simulink subsystem "slagEnergyBalance"  (R2024a)
settings: Solver=VariableStepAuto  StartTime=0.0  StopTime=2014080  RelTol=1e-3
undefined symbols (not defined in the file): bath_area, matte_specific_heat_capacity, slag_charge_heat_transfer_coefficient, slag_in_temperature, slag_matte_heat_transfer_coefficient, slag_specific_heat_capacity, water_specific_heat_capacity
settings Model: DataDictionary=constants.sldd  EnableAccessToBaseWorkspace=off  DefaultTestHarness=slagEnergyBalance_HarnessFromWorkspace  Creator=jason.miskin  LastModifiedBy=jason.miskin

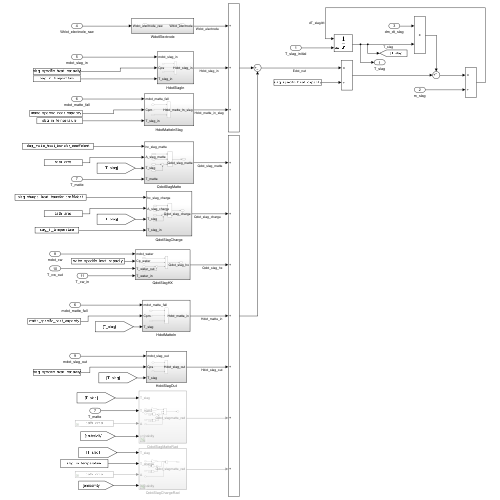
[thumbnail: Simulink's stored preview of the top-level diagram]
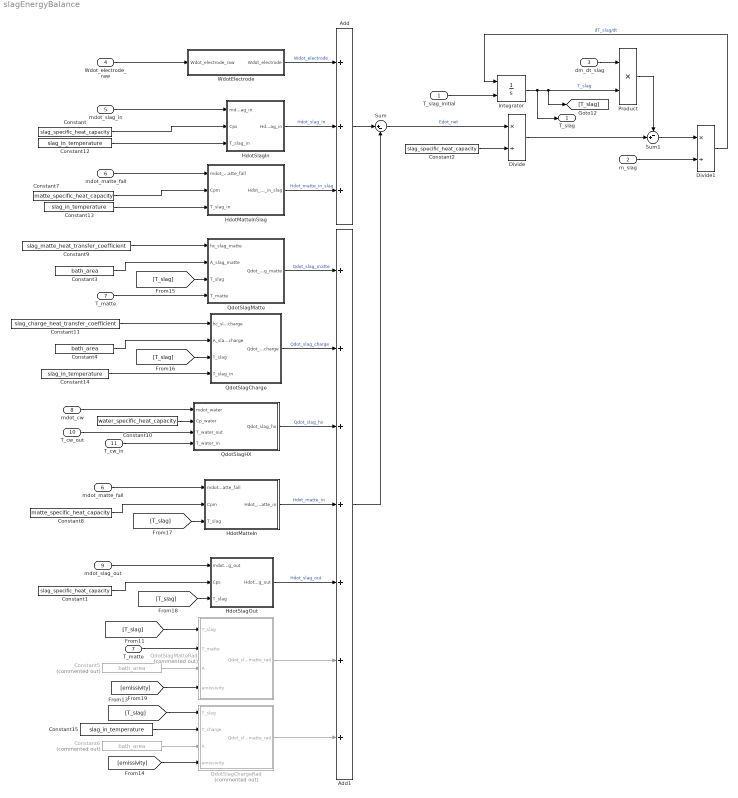
== system slagEnergyBalance ==
  T_slag_initial : Inport
  m_slag : Inport  Port=2
  dm_dt_slag : Inport  Port=3
  Wdot_electrode_raw : Inport  Port=4
  mdot_slag_in : Inport  Port=5
  mdot_matte_fall : Inport  Port=6
  T_matte : Inport  Port=7
  mdot_cw : Inport  Port=8
  mdot_slag_out : Inport  Port=9
  T_cw_out : Inport  Port=10
  T_cw_in : Inport  Port=11
  Add : Sum  Inputs=3
  Add1 : Sum  Inputs=7
  Constant : Constant  Value=slag_specific_heat_capacity
  Constant1 : Constant  Value=slag_specific_heat_capacity
  Constant10 : Constant  Value=water_specific_heat_capacity
  Constant11 : Constant  Value=slag_charge_heat_transfer_coefficient
  Constant{12..15} (4 alike) : Constant  Value=slag_in_temperature
  Constant2 : Constant  Value=slag_specific_heat_capacity
  Constant3 : Constant  Value=bath_area
  Constant4 : Constant  Value=bath_area
  Constant5 : Constant  Commented=on  Value=bath_area
  Constant6 : Constant  Commented=on  Value=bath_area
  Constant7 : Constant  Value=matte_specific_heat_capacity
  Constant8 : Constant  Value=matte_specific_heat_capacity
  Constant9 : Constant  Value=slag_matte_heat_transfer_coefficient
  Divide : Product  Inputs=*/
  Divide1 : Product  Inputs=*/
  HdotMatteIn : Subsystem
  HdotMatteInSlag : Subsystem
  HdotSlagIn : Subsystem
  HdotSlagOut : Subsystem
  Integrator : Integrator  InitialConditionSource=external
  Product : Product
  QdotSlagCharge : Subsystem
  QdotSlagChargeRad : Subsystem  Commented=on
  QdotSlagHX : Subsystem
  QdotSlagMatte : Subsystem
  QdotSlagMatteRad : Subsystem  Commented=on
  Sum : Sum  Inputs=|+-
  Sum1 : Sum  Inputs=-+|
  "T_matte " : InportShadow  Port=7
  WdotElectrode : Subsystem
  "mdot_matte_fall " : InportShadow  Port=6
  T_slag : Outport
  wires:
  WdotElectrode/1(Wdot_electrode) -> Add/1  "Wdot_electrode"
  Sum/1 -> Divide/1  "Edot_net"
  Constant/1 -> HdotSlagIn/2(Cps)
  [T_slag] -> HdotMatteIn/3(T_slag)
  Constant12/1 -> HdotSlagIn/3(T_slag_in)
  mdot_matte_fall/1 -> HdotMatteInSlag/1(mdot_matte_fall)
  T_slag_initial/1 -> Integrator/2
  Constant7/1 -> HdotMatteInSlag/2(Cpm)
  Divide/1 -> Sum1/2
  Constant3/1 -> QdotSlagMatte/2(A_slag_matte)
  mdot_slag_out/1 -> HdotSlagOut/1(mdot_slag_out)
  Divide1/1 -> Integrator/1  "dT_slag/dt"
  Constant9/1 -> QdotSlagMatte/1(hc_slag_matte)
  HdotSlagIn/1(Hdot_slag_in) -> Add/2  "Hdot_slag_in"
  dm_dt_slag/1 -> Product/1
  HdotMatteInSlag/1(Hdot_matte_in_slag) -> Add/3  "Hdot_matte_in_slag"
  HdotMatteIn/1(Hdot_matte_in) -> Add1/4  "Hdot_matte_in"
  Add/1 -> Sum/1
  QdotSlagMatte/1(Qdot_slag_matte) -> Add1/1  "Qdot_slag_matte"
  Integrator/1 -> Product/2, [T_slag], T_slag/1  "T_slag"
  Constant11/1 -> QdotSlagCharge/1(hc_slag_charge)
  m_slag/1 -> Divide1/2
  Add1/1 -> Sum/2
  Wdot_electrode_raw/1 -> WdotElectrode/1(Wdot_electrode_raw)
  QdotSlagCharge/1(Qdot_slag_charge) -> Add1/2  "Qdot_slag_charge"
  HdotSlagOut/1(Hdot_slag_out) -> Add1/5  "Hdot_slag_out"
  [T_slag] -> HdotSlagOut/3(T_slag)
  mdot_slag_in/1 -> HdotSlagIn/1(mdot_slag_in)
  Product/1 -> Sum1/1
  [T_slag] -> QdotSlagCharge/3(T_slag)
  [T_slag] -> QdotSlagMatte/3(T_slag)
  Sum1/1 -> Divide1/1
  mdot_cw/1 -> QdotSlagHX/1(mdot_water)
  QdotSlagHX/1(Qdot_slag_hx) -> Add1/3  "Qdot_slag_hx"
  T_matte/1 -> QdotSlagMatte/4(T_matte)
  Constant2/1 -> Divide/2
  Constant1/1 -> HdotSlagOut/2(Cps)
  Constant13/1 -> HdotMatteInSlag/3(T_slag_in)
  Constant14/1 -> QdotSlagCharge/4(T_slag_in)
  "mdot_matte_fall "/1 -> HdotMatteIn/1(mdot_matte_fall)
  Constant8/1 -> HdotMatteIn/2(Cpm)
  Constant4/1 -> QdotSlagCharge/2(A_slag_charge)
  T_cw_out/1 -> QdotSlagHX/3(T_water_out)
  T_cw_in/1 -> QdotSlagHX/4(T_water_in)
  Constant10/1 -> QdotSlagHX/2(Cp_water)
  Constant5/1 -> QdotSlagMatteRad/3(A)
  [T_slag] -> QdotSlagMatteRad/1(T_slag)
  "T_matte "/1 -> QdotSlagMatteRad/2(T_matte)
  Constant15/1 -> QdotSlagChargeRad/2(T_charge)
  Constant6/1 -> QdotSlagChargeRad/3(A)
  [T_slag] -> QdotSlagChargeRad/1(T_slag)
  QdotSlagMatteRad/1(Qdot_slagmatte_rad) -> Add1/6
  QdotSlagChargeRad/1(Qdot_slagmatte_rad) -> Add1/7
  [emissivity] -> QdotSlagChargeRad/4(emissivity)
  [emissivity] -> QdotSlagMatteRad/4(emissivity)

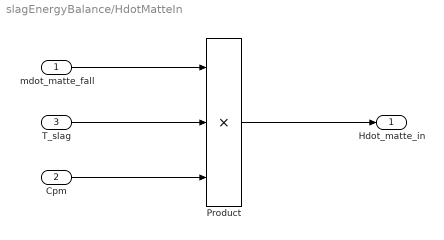
== system slagEnergyBalance/HdotMatteIn ==
  mdot_matte_fall : Inport
  Cpm : Inport  Port=2
  T_slag : Inport  Port=3
  Product : Product  Inputs=3
  Hdot_matte_in : Outport
  wires:
  T_slag/1 -> Product/2
  mdot_matte_fall/1 -> Product/1
  Product/1 -> Hdot_matte_in/1
  Cpm/1 -> Product/3

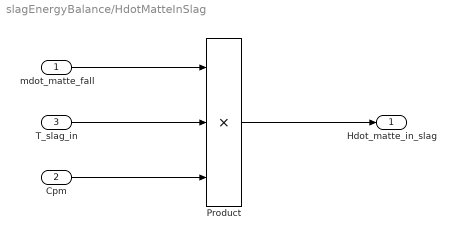
== system slagEnergyBalance/HdotMatteInSlag ==
  mdot_matte_fall : Inport
  Cpm : Inport  Port=2
  T_slag_in : Inport  Port=3
  Product : Product  Inputs=3
  Hdot_matte_in_slag : Outport
  wires:
  Cpm/1 -> Product/3
  mdot_matte_fall/1 -> Product/1
  Product/1 -> Hdot_matte_in_slag/1
  T_slag_in/1 -> Product/2

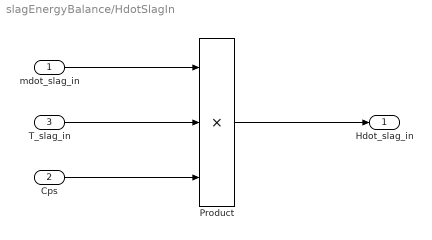
== system slagEnergyBalance/HdotSlagIn ==
  mdot_slag_in : Inport
  Cps : Inport  Port=2
  T_slag_in : Inport  Port=3
  Product : Product  Inputs=3
  Hdot_slag_in : Outport
  wires:
  Cps/1 -> Product/3
  T_slag_in/1 -> Product/2
  mdot_slag_in/1 -> Product/1
  Product/1 -> Hdot_slag_in/1

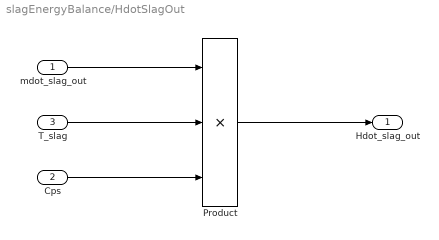
== system slagEnergyBalance/HdotSlagOut ==
  mdot_slag_out : Inport
  Cps : Inport  Port=2
  T_slag : Inport  Port=3
  Product : Product  Inputs=3
  Hdot_slag_out : Outport
  wires:
  Cps/1 -> Product/3
  mdot_slag_out/1 -> Product/1
  T_slag/1 -> Product/2
  Product/1 -> Hdot_slag_out/1

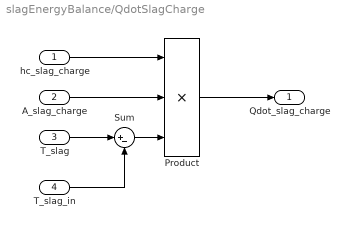
== system slagEnergyBalance/QdotSlagCharge ==
  hc_slag_charge : Inport
  A_slag_charge : Inport  Port=2
  T_slag : Inport  Port=3
  T_slag_in : Inport  Port=4
  Product : Product  Inputs=3
  Sum : Sum  Inputs=|+-
  Qdot_slag_charge : Outport
  wires:
  hc_slag_charge/1 -> Product/1
  A_slag_charge/1 -> Product/2
  T_slag/1 -> Sum/1
  T_slag_in/1 -> Sum/2
  Sum/1 -> Product/3
  Product/1 -> Qdot_slag_charge/1

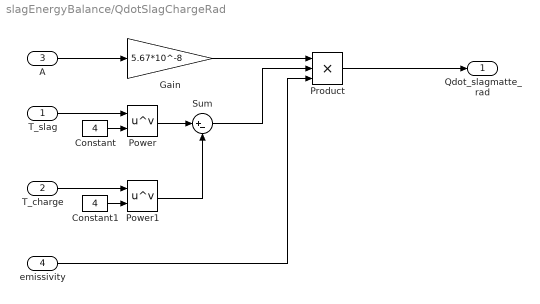
== system slagEnergyBalance/QdotSlagChargeRad ==
  T_slag : Inport
  T_charge : Inport  Port=2
  A : Inport  Port=3
  emissivity : Inport  Port=4
  Constant : Constant  Value=4
  Constant1 : Constant  Value=4
  Gain : Gain  Gain=5.67*10^-8
  Power : Math  Operator=pow
  Power1 : Math  Operator=pow
  Product : Product  Inputs=3
  Sum : Sum  Inputs=|+-
  Qdot_slagmatte_rad : Outport
  wires:
  emissivity/1 -> Product/3
  A/1 -> Gain/1
  T_slag/1 -> Power/1
  Constant/1 -> Power/2
  Constant1/1 -> Power1/2
  T_charge/1 -> Power1/1
  Gain/1 -> Product/1
  Product/1 -> Qdot_slagmatte_rad/1
  Power/1 -> Sum/1
  Power1/1 -> Sum/2
  Sum/1 -> Product/2

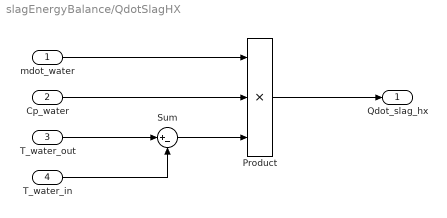
== system slagEnergyBalance/QdotSlagHX ==
  mdot_water : Inport
  Cp_water : Inport  Port=2
  T_water_out : Inport  Port=3
  T_water_in : Inport  Port=4
  Product : Product  Inputs=3
  Sum : Sum  Inputs=|+-
  Qdot_slag_hx : Outport
  wires:
  mdot_water/1 -> Product/1
  Product/1 -> Qdot_slag_hx/1
  Cp_water/1 -> Product/2
  T_water_in/1 -> Sum/2
  T_water_out/1 -> Sum/1
  Sum/1 -> Product/3

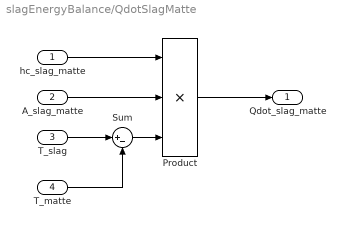
== system slagEnergyBalance/QdotSlagMatte ==
  hc_slag_matte : Inport
  A_slag_matte : Inport  Port=2
  T_slag : Inport  Port=3
  T_matte : Inport  Port=4
  Product : Product  Inputs=3
  Sum : Sum  Inputs=|+-
  Qdot_slag_matte : Outport
  wires:
  Product/1 -> Qdot_slag_matte/1
  Sum/1 -> Product/3
  T_matte/1 -> Sum/2
  T_slag/1 -> Sum/1
  A_slag_matte/1 -> Product/2
  hc_slag_matte/1 -> Product/1

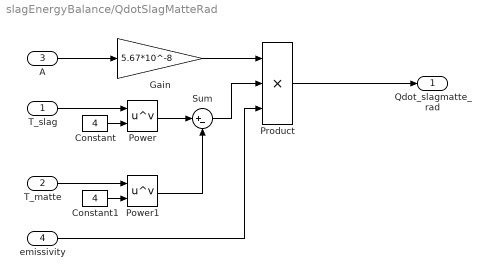
== system slagEnergyBalance/QdotSlagMatteRad ==
  T_slag : Inport
  T_matte : Inport  Port=2
  A : Inport  Port=3
  emissivity : Inport  Port=4
  Constant : Constant  Value=4
  Constant1 : Constant  Value=4
  Gain : Gain  Gain=5.67*10^-8
  Power : Math  Operator=pow
  Power1 : Math  Operator=pow
  Product : Product  Inputs=3
  Sum : Sum  Inputs=|+-
  Qdot_slagmatte_rad : Outport
  wires:
  emissivity/1 -> Product/3
  Sum/1 -> Product/2
  Power1/1 -> Sum/2
  Power/1 -> Sum/1
  Product/1 -> Qdot_slagmatte_rad/1
  Gain/1 -> Product/1
  T_matte/1 -> Power1/1
  Constant1/1 -> Power1/2
  Constant/1 -> Power/2
  T_slag/1 -> Power/1
  A/1 -> Gain/1

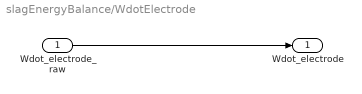
== system slagEnergyBalance/WdotElectrode ==
  Wdot_electrode_raw : Inport
  Wdot_electrode : Outport
  wires:
  Wdot_electrode_raw/1 -> Wdot_electrode/1
